simulink model "s_jsj4_70005"  (Simulink 5.0)
settings: Solver=ode45  SolverMode=SingleTasking  StartTime=0.0  StopTime=1  FixedStep=0.001  RelTol=1e-3
libraries: cstblocks x2
settings Model: LastModifiedBy=ThinkPad

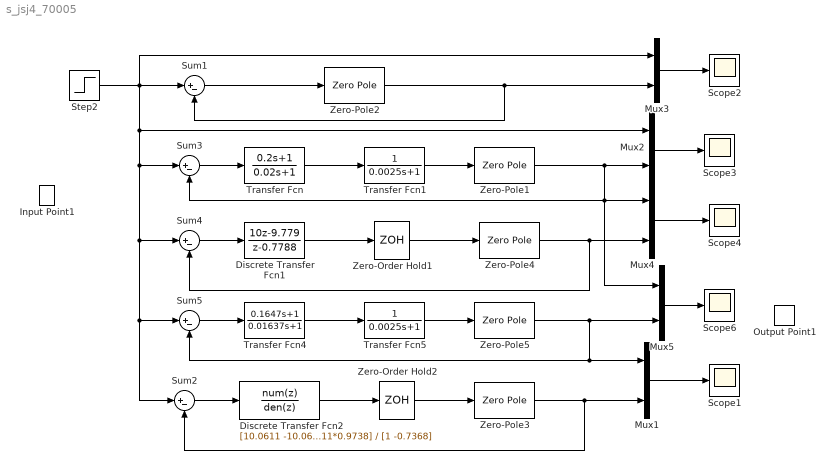
== system s_jsj4_70005 ==
  Discrete Transfer Fcn1 : DiscreteTransferFcn  Numerator=[10 -9.779]  Denominator=[1 -0.7788]  SampleTime=0.005
  Discrete Transfer Fcn2 : DiscreteTransferFcn  Numerator=[10.0611 -10.0611*0.9738]  Denominator=[1 -0.7368]  SampleTime=0.005
  Input Point1 : cstblocks/Input Point
  Mux{1..5} (5 alike) : Mux  Inputs=2
  Output Point1 : cstblocks/Output Point
  Scope{1..4,6} (5 alike) : Scope
      Scope1 settings: YMin=-3.5  YMax=1  MaxDataPoints=500000
      Scope2 settings: YMin=-3.5  YMax=1  MaxDataPoints=500000
      Scope3 settings: YMin=-3.5  YMax=1  SaveName=ScopeData2  MaxDataPoints=500000
      Scope4 settings: YMin=-3.5  YMax=1  SaveName=ScopeData3  MaxDataPoints=500000
      Scope6 settings: YMin=-3.5  YMax=1  SaveName=ScopeData5  MaxDataPoints=500000
  Step2 : Step  Time=0  SampleTime=0
  Sum{1..5} (5 alike) : Sum  Inputs=|+-  SaturateOnIntegerOverflow=on
  Transfer Fcn : TransferFcn  Numerator=[0.2 1]  Denominator=[0.02 1]
  Transfer Fcn1 : TransferFcn  Denominator=[0.0025 1]
  Transfer Fcn4 : TransferFcn  Numerator=[0.1647 1]  Denominator=[0.01637 1]
  Transfer Fcn5 : TransferFcn  Denominator=[0.0025 1]
  Zero-Order Hold1 : ZeroOrderHold  SampleTime=0.005
  Zero-Order Hold2 : ZeroOrderHold  SampleTime=0.005
  Zero-Pole{1..5} (5 alike) : ZeroPole  Zeros=[]  Poles=[0 -4]  Gain=[120]
  wires:
  Step2/1 -> Mux3/1, Sum1/1, Mux2/1, Sum3/1, Sum4/1, Sum5/1, Sum2/1
  Mux2/1 -> Scope3/1
  Zero-Pole1/1 -> Mux2/2, Sum3/2, Mux4/1, Mux5/1
  Transfer Fcn/1 -> Transfer Fcn1/1
  Transfer Fcn1/1 -> Zero-Pole1/1
  Mux3/1 -> Scope2/1
  Zero-Pole2/1 -> Mux3/2, Sum1/2
  Sum1/1 -> Zero-Pole2/1
  Sum3/1 -> Transfer Fcn/1
  Mux4/1 -> Scope4/1
  Zero-Pole4/1 -> Mux4/2, Sum4/2
  Discrete Transfer Fcn1/1 -> Zero-Order Hold1/1
  Sum4/1 -> Discrete Transfer Fcn1/1
  Zero-Order Hold1/1 -> Zero-Pole4/1
  Mux5/1 -> Scope6/1
  Zero-Pole5/1 -> Mux5/2, Mux1/1, Sum5/2
  Transfer Fcn4/1 -> Transfer Fcn5/1
  Transfer Fcn5/1 -> Zero-Pole5/1
  Sum5/1 -> Transfer Fcn4/1
  Mux1/1 -> Scope1/1
  Zero-Pole3/1 -> Mux1/2, Sum2/2
  Discrete Transfer Fcn2/1 -> Zero-Order Hold2/1
  Sum2/1 -> Discrete Transfer Fcn2/1
  Zero-Order Hold2/1 -> Zero-Pole3/1
